simulink model "pmsm_speed_control"  (R2024b)
settings: Solver=VariableStepAuto  StartTime=0.0  StopTime=10.0  RelTol=1e-3
values from neighbouring files (symbols this model uses):
  Iq_max = 120    [step3_build_speed_loop.m]    (also in step4_build_position_loop.m; step5b_current_control.m; step5c_speed_control.m; step5d_position_control.m)
  Ki_speed = 1.5    [simulate_surface_pmsm_foc.m]    (also in step3_build_speed_loop.m = 2 * pi * f_bw_speed * motor.B / k_torque; step4_build_position_loop.m = 2 * pi * f_bw_speed * motor.B / k_torque; step5c_speed_control.m = 0.523598775598; step5d_position_control.m = 0.523598775598)
  Kp_speed = 0.15    [simulate_surface_pmsm_foc.m]    (also in step3_build_speed_loop.m = 2 * pi * f_bw_speed * motor.J / k_torque; step4_build_position_loop.m = 2 * pi * f_bw_speed * motor.J / k_torque; step5c_speed_control.m = 5.23598775598; step5d_position_control.m = 5.23598775598)
settings Model: Creator=Lee  LastModifiedBy=Lee

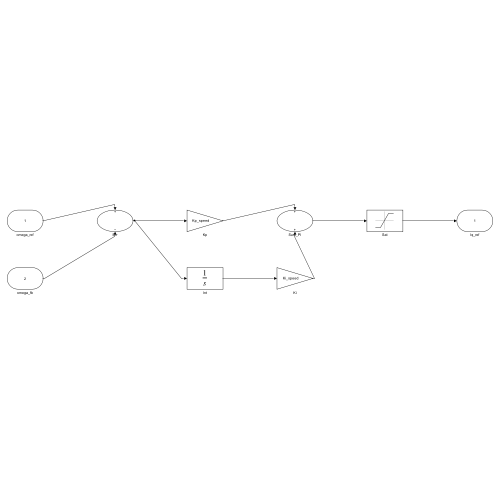
[thumbnail: Simulink's stored preview of the top-level diagram]
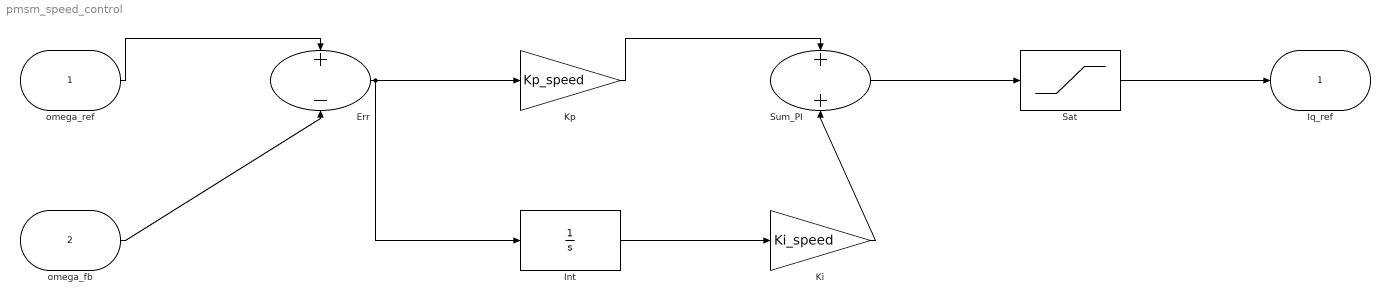
== system pmsm_speed_control ==
  omega_ref : Inport
  omega_fb : Inport  Port=2
  Err : Sum  Inputs=+-
  Int : Integrator
  Ki : Gain  Gain=Ki_speed
  Kp : Gain  Gain=Kp_speed
  Sat : Saturate  UpperLimit=Iq_max  LowerLimit=-Iq_max
  Sum_PI : Sum
  Iq_ref : Outport
  wires:
  omega_ref/1 -> Err/1
  omega_fb/1 -> Err/2
  Err/1 -> Kp/1, Int/1
  Int/1 -> Ki/1
  Kp/1 -> Sum_PI/1
  Ki/1 -> Sum_PI/2
  Sum_PI/1 -> Sat/1
  Sat/1 -> Iq_ref/1
